simulink model "adaptive_mrac_e2y_double_delay"  (R2020a)
settings: Solver=FixedStepAuto  StartTime=0.0  StopTime=89.99  FixedStep=0.01  RelTol=1e-3
values from neighbouring files (symbols this model uses):
  gamma_x = [0.5; 0.5]    [cases_test.m]    (also in cases_tests_lr.m = gamma_x_0 * i; mrac_model_const_ref.m = params(4:5); mrac_model_e2y.m = params(5:6); mrac_model_e2y_2delay.m = params(7:8))
  k_x0 = k_x0_list(:, plant_case)    [cases_test.m]    (also in mrac_model_const_ref.m = [-params(1); params(2)]; mrac_model_e2y.m = params(1:2); mrac_model_e2y_2delay.m = params(1:2); mrac_model_lr_init.m = [-params(1); params(2)])
  P = lyap(ref_sys.A', eye(2))    [cases_test.m]    (also in cases_tests_lr.m; mrac_model_e2y.m = [1.5 1; 1.5, 1]; mrac_model_e2y_2delay.m = [1.5, 3; 1.5, 3]; mrac_model_lr_init_low_pass_comp.m = params(3:4))
  ref_sys = canon(ref_sys, 'modal')    [cases_test.m]    (also in cases_tests_lr.m; mrac_model.m = ss([tf_cl_pade; s*tf_cl_pade]); mrac_model_e2y.m = ss([tf_cl_pade; s*tf_cl_pade]); mrac_model_e2y_2delay.m = ss([tf_cl_pade; s*tf_cl_pade]))
  tau_0 = params(9)    [mrac_model_e2y_2delay.m]
undefined symbols (not defined in the file or in its folder): case_, ref_x0, tau_d, tau_p
libraries: commfilt2 x2, dspstat3 x1
settings Model: OrderedModelArguments=off  Creator=lorenzoterenzi  LastModifiedBy=lorenzoterenzi

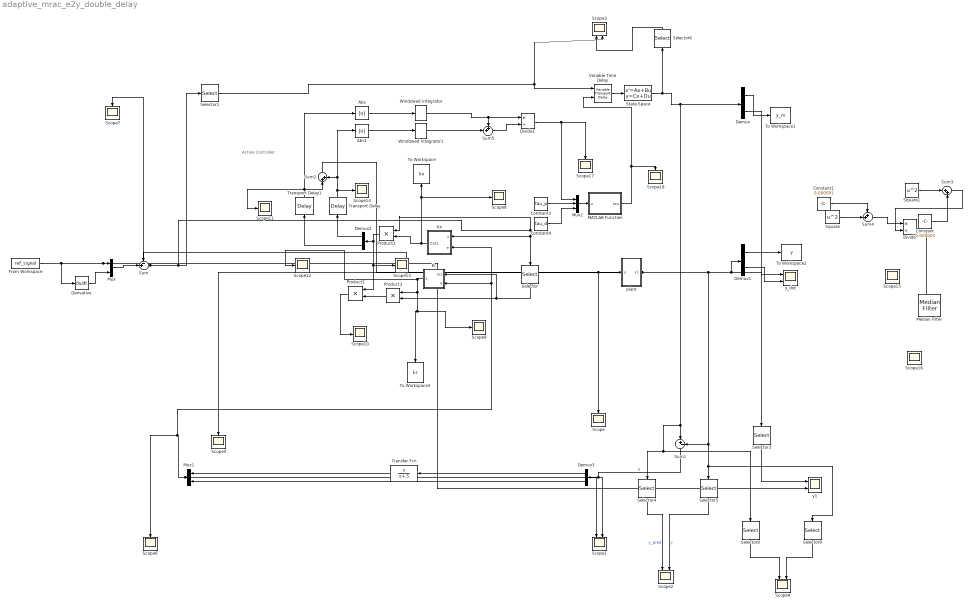
== system adaptive_mrac_e2y_double_delay ==
  note: Active Controller
  Abs : Abs
  Abs1 : Abs
  Constant : Constant  Value=0.000001
  Constant1 : Constant  Value=0.000001
  Constant3 : Constant  Value=tau_p
  Constant4 : Constant  Value=tau_d
  Demux{,1..3} (4 alike) : Demux  Outputs=2
  Derivative : Derivative
  Divide : Product  Inputs=*/
  Divide1 : Product  Inputs=*/
  From Workspace : FromWorkspace  VariableName=ref_signal
  Kr : Subsystem
  Kx : Subsystem
  MATLAB Function : MATLAB Function  TreatAsAtomicUnit=on
  Median Filter : dspstat3/Median Filter  WindowLength=5  SimulateUsing=Code generation
      settings: SourceProductBaseCode=DS
  Mux : Mux  Inputs=2
  Mux1 : Mux  Inputs=2
  Mux2 : Mux  Inputs=3
  Product1 : Product
  Product2 : Product
  Product3 : Product
  Scope{,5..18} (15 alike) : Scope
  Scope{1..4} (4 alike) : Scope  NumInputPorts=2
  Selector : Selector  InputPortWidth=2  IndexOptions=Index vector (dialog)  Indices=[2]  OutputSizes=1
  Selector{1,3..6} (5 alike) : Selector  InputPortWidth=2  IndexOptions=Index vector (dialog)  Indices=[1]  OutputSizes=1
  Selector8 : Selector  InputPortWidth=2  IndexOptions=Index vector (dialog)  Indices=[2]  OutputSizes=1
  Selector9 : Selector  InputPortWidth=2  IndexOptions=Index vector (dialog)  Indices=[2]  OutputSizes=1
  Square : Math  Operator=square  SaturateOnIntegerOverflow=on
  Square1 : Math  Operator=square  SaturateOnIntegerOverflow=on
  State-Space : StateSpace  A=ref_sys.A  B=ref_sys.B  C=ref_sys.C  D=ref_sys.D  InitialCondition=ref_x0
  Sum : Sum  Inputs=-+|
  Sum1 : Sum  Inputs=|+-
  Sum2 : Sum  Inputs=|++
  Sum3 : Sum  Inputs=|++
  Sum4 : Sum  Inputs=++|
  Sum5 : Sum  Inputs=++|
  To Workspace : ToWorkspace  VariableName=kx  SaveFormat=Timeseries  SampleTime=-1
  To Workspace1 : ToWorkspace  VariableName=y_m  SaveFormat=Timeseries  SampleTime=-1
  To Workspace2 : ToWorkspace  VariableName=y  SaveFormat=Timeseries  SampleTime=-1
  To Workspace3 : ToWorkspace  VariableName=kr  SaveFormat=Timeseries  SampleTime=-1
  Transfer Fcn : TransferFcn  Numerator=[1 0]  Denominator=[1 .5]
  Transport Delay : TransportDelay  DelayTime=tau_p
  Transport Delay1 : TransportDelay  DelayTime=tau_d
  Variable Time Delay : VariableTransportDelay  MaximumDelay=10
  Windowed Integrator : commfilt2/Windowed Integrator  integperiod=500  InputProcessing=Columns as channels (frame based)  roundingMode=Floor  overflowMode=off  coeffDataTypeStr=Inherit: Same word length as input  coeffMin=[]  coeffMax=[]  coeffLastDataTypeStr=Inherit: Same word length as input  accumDataTypeStr=Inherit: Same as product output  accumLastDataTypeStr=Inherit: Same as product output  outputDataTypeStr=Inherit: Same as accumulator  outputMin=[]  outputMax=[]  outputLastDataTypeStr=Inherit: Same as accumulator
      settings: SourceProductBaseCode=CM
  Windowed Integrator1 : commfilt2/Windowed Integrator  integperiod=500  InputProcessing=Columns as channels (frame based)  roundingMode=Floor  overflowMode=off  coeffDataTypeStr=Inherit: Same word length as input  coeffMin=[]  coeffMax=[]  coeffLastDataTypeStr=Inherit: Same word length as input  accumDataTypeStr=Inherit: Same as product output  accumLastDataTypeStr=Inherit: Same as product output  outputDataTypeStr=Inherit: Same as accumulator  outputMin=[]  outputMax=[]  outputLastDataTypeStr=Inherit: Same as accumulator
      settings: SourceProductBaseCode=CM
  plant : Subsystem
  y1 : Scope  NumInputPorts=2
  y_dot : Scope  NumInputPorts=2
  wires:
  Demux/2 -> y_dot/1
  Sum1/1 -> Demux3/1, Scope1/2  "e"
  Demux1/2 -> y_dot/2
  Demux/1 -> To Workspace1/1
  State-Space/1 -> Demux/1, Selector4/1, Selector8/1, Sum1/1, Selector6/1
  Demux1/1 -> To Workspace2/1
  Sum2/1 -> plant/1(u), Scope/1
  Selector3/1 -> y1/1
  Selector4/1 -> Scope2/1  "y_pred"
  Selector5/1 -> Scope2/2  "y"
  Selector6/1 -> Scope3/1
  Selector8/1 -> Scope4/1
  Selector9/1 -> Scope4/2
  plant/1(x1) -> Scope5/1, Sum/1, Demux1/1, Selector3/1, Sum1/2, Selector9/1, Selector5/1
  Selector1/1 -> Variable Time Delay/1, Scope3/2
  From Workspace/1 -> y1/2, Mux/1, Derivative/1
  Mux/1 -> Sum/2
  Derivative/1 -> Mux/2
  Demux3/1 -> Transfer Fcn/1
  Demux3/2 -> Mux1/2
  Transfer Fcn/1 -> Mux1/1
  Variable Time Delay/1 -> State-Space/1
  Transport Delay1/1 -> Abs/1, Sum2/1, Scope11/1
  Demux2/1 -> Transport Delay/1
  Demux2/2 -> Transport Delay1/1
  Transport Delay/1 -> Scope14/1, Abs1/1, Sum2/2
  Sum/1 -> Product2/1, Kx/1(x), Selector/1, Selector1/1, Scope7/1
  Product3/1 -> Product1/2
  Mux1/1 -> Kx/2(e), Kr/2(e), Scope6/1, Scope1/1
  Selector/1 -> Kr/1(In1), Product3/2
  Kr/1(Out1) -> Scope12/1, Product3/1, To Workspace3/1, Scope9/1
  Product1/1 -> Scope10/1
  Product2/1 -> Demux2/1, Scope13/1, Product1/1
  Kx/1(Out1) -> Product2/2, To Workspace/1, Scope8/1
  Square1/1 -> Sum3/1
  Square/1 -> Sum4/2
  Sum4/1 -> Divide/1
  Sum3/1 -> Divide/2
  Constant/1 -> Sum3/2
  Constant1/1 -> Sum4/1
  MATLAB Function/1(tau) -> Scope18/1, Variable Time Delay/2
  Divide/1 -> Median Filter/1
  Windowed Integrator/1 -> Sum5/1, Divide1/1
  Divide1/1 -> Mux2/1, Scope17/1
  Abs/1 -> Windowed Integrator/1
  Abs1/1 -> Windowed Integrator1/1
  Windowed Integrator1/1 -> Sum5/2
  Sum5/1 -> Divide1/2
  Mux2/1 -> MATLAB Function/1(u)
  Constant3/1 -> Mux2/2
  Constant4/1 -> Mux2/3

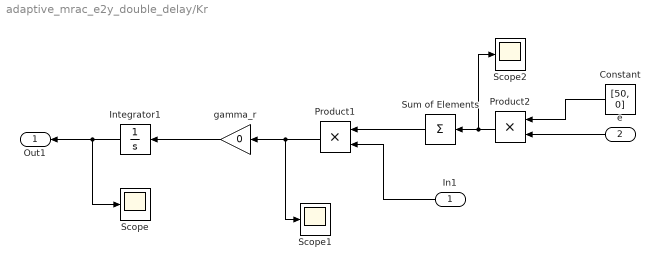
== system adaptive_mrac_e2y_double_delay/Kr ==
  In1 : Inport
  e : Inport  Port=2
  Constant : Constant  Value=[50, 0]
  Integrator1 : Integrator  InitialCondition=tau_0
  Product1 : Product
  Product2 : Product
  Scope : Scope
  Scope1 : Scope
  Scope2 : Scope
  Sum of Elements : Sum  Inputs=+
  gamma_r : Gain  Gain=0
  Out1 : Outport
  wires:
  In1/1 -> Product1/2
  Product1/1 -> Scope1/1, gamma_r/1
  Product2/1 -> Scope2/1, Sum of Elements/1
  e/1 -> Product2/2
  Sum of Elements/1 -> Product1/1
  Integrator1/1 -> Out1/1, Scope/1
  Constant/1 -> Product2/1
  gamma_r/1 -> Integrator1/1

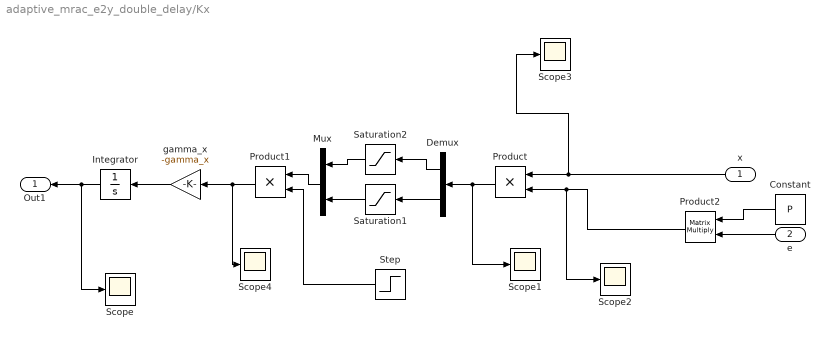
== system adaptive_mrac_e2y_double_delay/Kx ==
  x : Inport
  e : Inport  Port=2
  Constant : Constant  Value=P
  Demux : Demux  Outputs=2
  Integrator : Integrator  InitialCondition=k_x0
  Mux : Mux  Inputs=2
  Product : Product
  Product1 : Product
  Product2 : Product  Multiplication=Matrix(*)
  Saturation1 : Saturate  UpperLimit=0.05  LowerLimit=-0.05
  Saturation2 : Saturate  UpperLimit=0.01  LowerLimit=-0.01
  Scope{,1..4} (5 alike) : Scope
  Step : Step  Time=20  SampleTime=0
  gamma_x : Gain  Gain=-gamma_x
  Out1 : Outport  PortDimensions=[2, 1]
  wires:
  x/1 -> Scope3/1, Product/1
  e/1 -> Product2/2
  Integrator/1 -> Scope/1, Out1/1
  Constant/1 -> Product2/1
  gamma_x/1 -> Integrator/1
  Product2/1 -> Scope2/1, Product/2
  Saturation1/1 -> Mux/2
  Demux/2 -> Saturation1/1
  Saturation2/1 -> Mux/1
  Demux/1 -> Saturation2/1
  Product/1 -> Scope1/1, Demux/1
  Product1/1 -> Scope4/1, gamma_x/1
  Mux/1 -> Product1/1
  Step/1 -> Product1/2

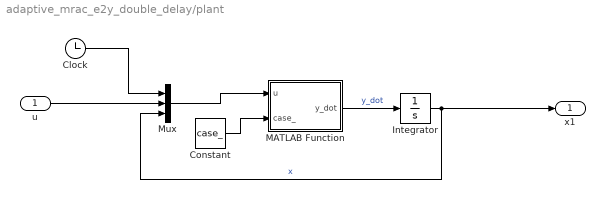
== system adaptive_mrac_e2y_double_delay/plant ==
  u : Inport
  Clock : Clock
  Constant : Constant  Value=case_
  Integrator : Integrator  InitialCondition=[0;0]
  MATLAB Function : MATLAB Function  TreatAsAtomicUnit=on
  Mux : Mux  Inputs=3
  x1 : Outport
  wires:
  Mux/1 -> MATLAB Function/1(u)
  Integrator/1 -> x1/1, Mux/3  "x"
  MATLAB Function/1(y_dot) -> Integrator/1  "y_dot"
  Clock/1 -> Mux/1
  Constant/1 -> MATLAB Function/2(case_)
  u/1 -> Mux/2

== matlab function adaptive_mrac_e2y_double_delay/plant/MATLAB Function ==
  data: u input size=4; y_dot output size=2; case_ input
function y_dot = fcn(u, case_)
    t = u(1);
    u_c = u(2);
    y_prev = u(3:4);
    y_dot = models.peter_plant(case_, t, u_c, y_prev);
end


% function y_dot = peter_plant(case_, t, u, y_prev)
%     % case 1: first to second order system transition
%     if case_ == 1
%         M = -1;
%         G = -100;
%     % case 2: second to first order transition
%     elseif case_ == 2 
%         M = 91;
%         G = 100;
%     elseif case_ == 3    
%         M = 50;
%         G = 0.5;
%     elseif case_ == 4
%         M = 50;
%         G = 100;
%     else
%         G = 0;
%         M = 0;
%     end
% 
%     omega_b1 = 6;
%     omega_b2 = 0.2;
%     k_c1 = 90;
%     k_c2 = 30;
% 
%     omega_b = omega_b1 + (omega_b2 - omega_b1)./(1 + exp(-G * (t - M)));
%     k_c = k_c1 + (k_c2 - k_c1)./(1 + exp(-G * (t - M)));
% 
%     A = [0, 1; 0, omega_b];
%     B = [0; k_c];
%     y_dot = A*y_prev + B*u;
% end

== matlab function adaptive_mrac_e2y_double_delay/MATLAB Function ==
  data: u input; tau output
function tau = fcn(u)
    weight = u(1);
    tau_p = u(2);
    tau_d = u(3);
    tau = weight * (tau_d - tau_p) + tau_p;
end
